simulink model "Part10"  (R2017b)
settings: Solver=VariableStepAuto  StartTime=0.0  StopTime=100  RelTol=1e-3
settings Model: Creator=Yazdanpanah  LastModifiedBy=admin
settings DataIOCC: ReturnWorkspaceOutputs=on
settings SFSimCC: SimUseLocalCustomCode=on
settings RTWCC: RTWUseLocalCustomCode=on
settings CodeAppCC: StateflowObjectComments=on

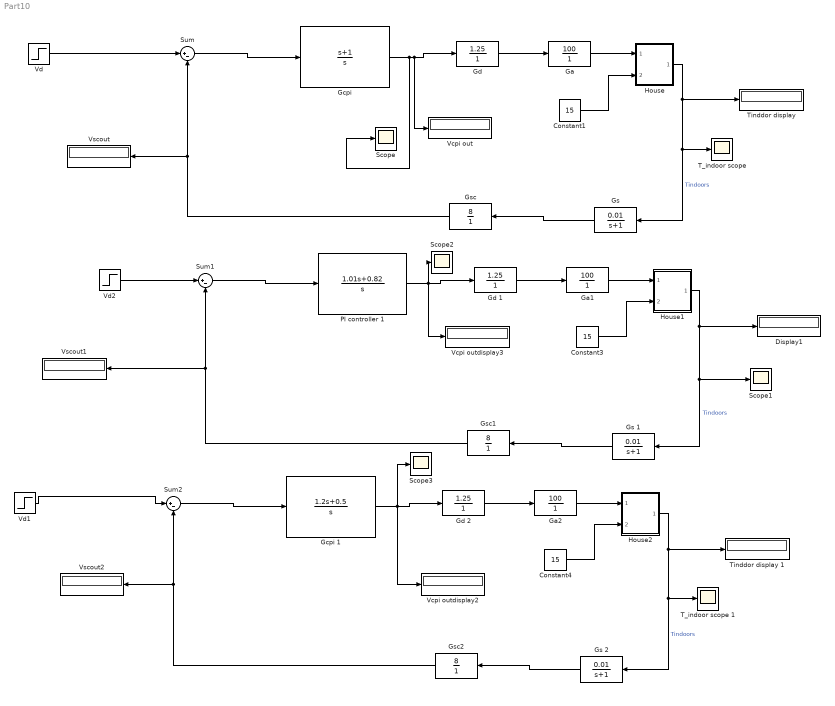
== system Part10 ==
  Constant1 : Constant  Value=15
  Constant3 : Constant  Value=15
  Constant4 : Constant  Value=15
  Display1 : Display
  Ga : TransferFcn  Numerator=[100]  Denominator=[1 ]
  Ga1 : TransferFcn  Numerator=[100]  Denominator=[1 ]
  Ga2 : TransferFcn  Numerator=[100]  Denominator=[1 ]
  "Gcpi " : TransferFcn  Numerator=[1 1]  Denominator=[1 0]
  Gcpi 1 : TransferFcn  Numerator=[1.2 0.5]  Denominator=[1 0]
  "Gd " : TransferFcn  Numerator=[1.25]  Denominator=[1 ]
  Gd 1 : TransferFcn  Numerator=[1.25]  Denominator=[1 ]
  Gd 2 : TransferFcn  Numerator=[1.25]  Denominator=[1 ]
  "Gs " : TransferFcn  Numerator=[0.01]  Denominator=[1 1]
  Gs 1 : TransferFcn  Numerator=[0.01]  Denominator=[1 1]
  Gs 2 : TransferFcn  Numerator=[0.01]  Denominator=[1 1]
  Gsc : TransferFcn  Numerator=[8]  Denominator=[1 ]
  Gsc1 : TransferFcn  Numerator=[8]  Denominator=[1 ]
  Gsc2 : TransferFcn  Numerator=[8]  Denominator=[1 ]
  House : Subsystem
      mask Display: image(fullfile(matlabroot,'toolbox','simulink','simdemos','simgeneral','images','HouseHeatHousePix.svg'))
  House1 : Subsystem
      mask Display: image(fullfile(matlabroot,'toolbox','simulink','simdemos','simgeneral','images','HouseHeatHousePix.svg'))
  House2 : Subsystem
      mask Display: image(fullfile(matlabroot,'toolbox','simulink','simdemos','simgeneral','images','HouseHeatHousePix.svg'))
  PI controller 1 : TransferFcn  Numerator=[1.01 0.82]  Denominator=[1 0]
  Scope{,1..3} (4 alike) : Scope
  Sum : Sum  Inputs=|+-
  Sum1 : Sum  Inputs=|+-
  Sum2 : Sum  Inputs=|+-
  "T_indoor scope " : Scope
  T_indoor scope 1 : Scope
  "Tinddor display " : Display
  Tinddor display 1 : Display
  Vcpi out : Display
  "Vcpi outdisplay2 " : Display
  "Vcpi outdisplay3 " : Display
  Vd : Step  Time=0  After=2.06  SampleTime=0
  Vd1 : Step  Time=0  After=2.06  SampleTime=0
  Vd2 : Step  Time=0  After=2.06  SampleTime=0
  Vscout : Display
  "Vscout1 " : Display
  Vscout2 : Display
  wires:
  Constant1/1 -> House/2(Outdoor Temp Tout)
  Sum/1 -> "Gcpi "/1
  "Gcpi "/1 -> Scope/1, Vcpi out/1, "Gd "/1
  "Gd "/1 -> Ga/1
  Ga/1 -> House/1(Heater QDot In)
  House/1(Room Temp Troom) -> "Tinddor display "/1, "T_indoor scope "/1, "Gs "/1  "Tindoors"
  "Gs "/1 -> Gsc/1
  Gsc/1 -> Vscout/1, Sum/2
  Gs 1/1 -> Gsc1/1
  House1/1(Room Temp Troom) -> Display1/1, Scope1/1, Gs 1/1  "Tindoors"
  Sum1/1 -> PI controller 1/1
  PI controller 1/1 -> "Vcpi outdisplay3 "/1, Scope2/1, Gd 1/1
  Ga1/1 -> House1/1(Heater QDot In)
  Gd 1/1 -> Ga1/1
  Gsc1/1 -> "Vscout1 "/1, Sum1/2
  Constant3/1 -> House1/2(Outdoor Temp Tout)
  Vd/1 -> Sum/1
  Vd1/1 -> Sum2/1
  Gs 2/1 -> Gsc2/1
  House2/1(Room Temp Troom) -> Tinddor display 1/1, T_indoor scope 1/1, Gs 2/1  "Tindoors"
  Sum2/1 -> Gcpi 1/1
  Gcpi 1/1 -> Scope3/1, "Vcpi outdisplay2 "/1, Gd 2/1
  Ga2/1 -> House2/1(Heater QDot In)
  Gd 2/1 -> Ga2/1
  Gsc2/1 -> Vscout2/1, Sum2/2
  Constant4/1 -> House2/2(Outdoor Temp Tout)
  Vd2/1 -> Sum1/1

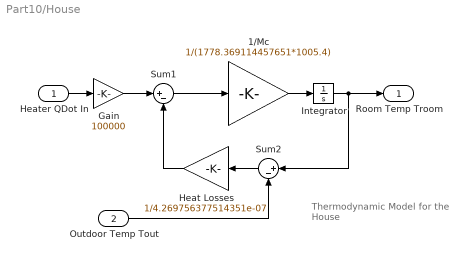
== system Part10/House ==
  note: Thermodynamic Model
      | for the House
  Heater QDot In : Inport
  Outdoor Temp Tout : Inport  Port=2
  1/Mc : Gain  Gain=1/(1778.369114457651*1005.4)  SaturateOnIntegerOverflow=on  OutDataTypeStr=Inherit: Same as input  ParamDataTypeStr=Inherit: Same as input
  Gain : Gain  Gain=100000
  Heat Losses : Gain  Gain=1/4.269756377514351e-07  SaturateOnIntegerOverflow=on  OutDataTypeStr=Inherit: Same as input  ParamDataTypeStr=Inherit: Same as input
  Integrator : Integrator  InitialCondition=20
  Sum1 : Sum  Inputs=|+-  SaturateOnIntegerOverflow=on  InputSameDT=on  OutDataTypeStr=Inherit: Same as first input
  Sum2 : Sum  Inputs=|+-  SaturateOnIntegerOverflow=on  InputSameDT=on  OutDataTypeStr=Inherit: Same as first input
  Room Temp Troom : Outport  InitialOutput=0
  wires:
  Outdoor Temp Tout/1 -> Sum2/2
  Heater QDot In/1 -> Gain/1
  Sum1/1 -> 1/Mc/1
  Sum2/1 -> Heat Losses/1
  Heat Losses/1 -> Sum1/2
  1/Mc/1 -> Integrator/1
  Integrator/1 -> Sum2/1, Room Temp Troom/1
  Gain/1 -> Sum1/1

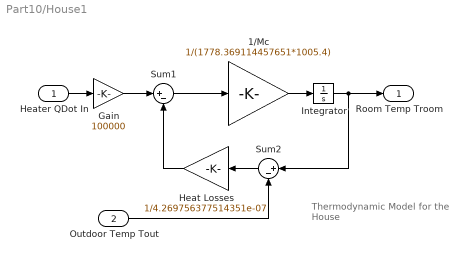
== system Part10/House1 ==
  note: Thermodynamic Model
      | for the House
  Heater QDot In : Inport
  Outdoor Temp Tout : Inport  Port=2
  1/Mc : Gain  Gain=1/(1778.369114457651*1005.4)  SaturateOnIntegerOverflow=on  OutDataTypeStr=Inherit: Same as input  ParamDataTypeStr=Inherit: Same as input
  Gain : Gain  Gain=100000
  Heat Losses : Gain  Gain=1/4.269756377514351e-07  SaturateOnIntegerOverflow=on  OutDataTypeStr=Inherit: Same as input  ParamDataTypeStr=Inherit: Same as input
  Integrator : Integrator  InitialCondition=20
  Sum1 : Sum  Inputs=|+-  SaturateOnIntegerOverflow=on  InputSameDT=on  OutDataTypeStr=Inherit: Same as first input
  Sum2 : Sum  Inputs=|+-  SaturateOnIntegerOverflow=on  InputSameDT=on  OutDataTypeStr=Inherit: Same as first input
  Room Temp Troom : Outport  InitialOutput=0
  wires:
  Outdoor Temp Tout/1 -> Sum2/2
  Heater QDot In/1 -> Gain/1
  Sum1/1 -> 1/Mc/1
  Sum2/1 -> Heat Losses/1
  Heat Losses/1 -> Sum1/2
  1/Mc/1 -> Integrator/1
  Integrator/1 -> Sum2/1, Room Temp Troom/1
  Gain/1 -> Sum1/1

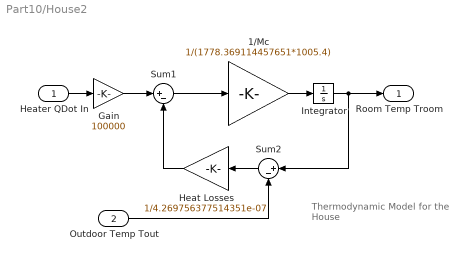
== system Part10/House2 ==
  note: Thermodynamic Model
      | for the House
  Heater QDot In : Inport
  Outdoor Temp Tout : Inport  Port=2
  1/Mc : Gain  Gain=1/(1778.369114457651*1005.4)  SaturateOnIntegerOverflow=on  OutDataTypeStr=Inherit: Same as input  ParamDataTypeStr=Inherit: Same as input
  Gain : Gain  Gain=100000
  Heat Losses : Gain  Gain=1/4.269756377514351e-07  SaturateOnIntegerOverflow=on  OutDataTypeStr=Inherit: Same as input  ParamDataTypeStr=Inherit: Same as input
  Integrator : Integrator  InitialCondition=20
  Sum1 : Sum  Inputs=|+-  SaturateOnIntegerOverflow=on  InputSameDT=on  OutDataTypeStr=Inherit: Same as first input
  Sum2 : Sum  Inputs=|+-  SaturateOnIntegerOverflow=on  InputSameDT=on  OutDataTypeStr=Inherit: Same as first input
  Room Temp Troom : Outport  InitialOutput=0
  wires:
  Outdoor Temp Tout/1 -> Sum2/2
  Heater QDot In/1 -> Gain/1
  Sum1/1 -> 1/Mc/1
  Sum2/1 -> Heat Losses/1
  Heat Losses/1 -> Sum1/2
  1/Mc/1 -> Integrator/1
  Integrator/1 -> Sum2/1, Room Temp Troom/1
  Gain/1 -> Sum1/1
